simulink model "neupravljani_nelinearni_i_linearni_model"  (R2015a)
settings: Solver=ode4  StartTime=0.0  StopTime=700  FixedStep=0.01  RelTol=1e-3
values from neighbouring files (symbols this model uses):
  Ar1 = 0.04    [skript_drugi_deo.m]
  Ar2 = 0.04    [skript_drugi_deo.m]
  Cd1 = 0.65    [skript_drugi_deo.m]
  Cd2 = 0.65    [skript_drugi_deo.m]
  Cdh = 0.65    [skript_drugi_deo.m]
  df1_H1 = double(subs(df1_H1, [Uvh Uv2 H1 H2], [Uvh_N Uv2_N H1_N H2_N]))    [skript_drugi_deo.m]
  df1_Uvh = double(subs(df1_Uvh, [Uvh Uv2 H1 H2], [Uvh_N Uv2_N H1_N H2_N]))    [skript_drugi_deo.m]
  df2_H1 = double(subs(df2_H1, [Uvh Uv2 H1 H2], [Uvh_N Uv2_N H1_N H2_N]))    [skript_drugi_deo.m]
  df2_H2 = double(subs(df2_H2, [Uvh Uv2 H1 H2], [Uvh_N Uv2_N H1_N H2_N]))    [skript_drugi_deo.m]
  df2_Uv2 = double(subs(df2_Uv2, [Uvh Uv2 H1 H2], [Uvh_N Uv2_N H1_N H2_N]))    [skript_drugi_deo.m]
  g = 9.81    [skript_drugi_deo.m]
  H1_max = 1.5    [skript_drugi_deo.m]
  H1_min = 0    [skript_drugi_deo.m]
  H1_N = 0.7    [skript_drugi_deo.m]
  H2_max = 1.5    [skript_drugi_deo.m]
  H2_min = 0    [skript_drugi_deo.m]
  H2_N = 0.8    [skript_drugi_deo.m]
  Kv1 = 1.5/1000    (= 0.0015)    [skript_drugi_deo.m]
  Kv2 = 1.5/1000    (= 0.0015)    [skript_drugi_deo.m]
  Kvh = 1/1000    (= 0.001)    [skript_drugi_deo.m]
  Ph = 3.25*10^5    (= 325000)    [skript_drugi_deo.m]
  ro = 1000    [skript_drugi_deo.m]
  Uv1 = 3    [skript_drugi_deo.m]
  Uv2_max = 10    [skript_drugi_deo.m]
  Uv2_min = 0    [skript_drugi_deo.m]
  Uv2_N = double(solve(e2 == 0, U2_N))    [skript_drugi_deo.m]
  Uvh_max = 10    [skript_drugi_deo.m]
  Uvh_min = 0    [skript_drugi_deo.m]
  Uvh_N = double(solve(e1 == 0, Uh_N))    [skript_drugi_deo.m]
  w1 = 0.1    [skript_drugi_deo.m]
  w2 = 0.1    [skript_drugi_deo.m]
  wh = 0.03    [skript_drugi_deo.m]
settings Model: Creator=Nikola  LastModifiedBy=Nikola

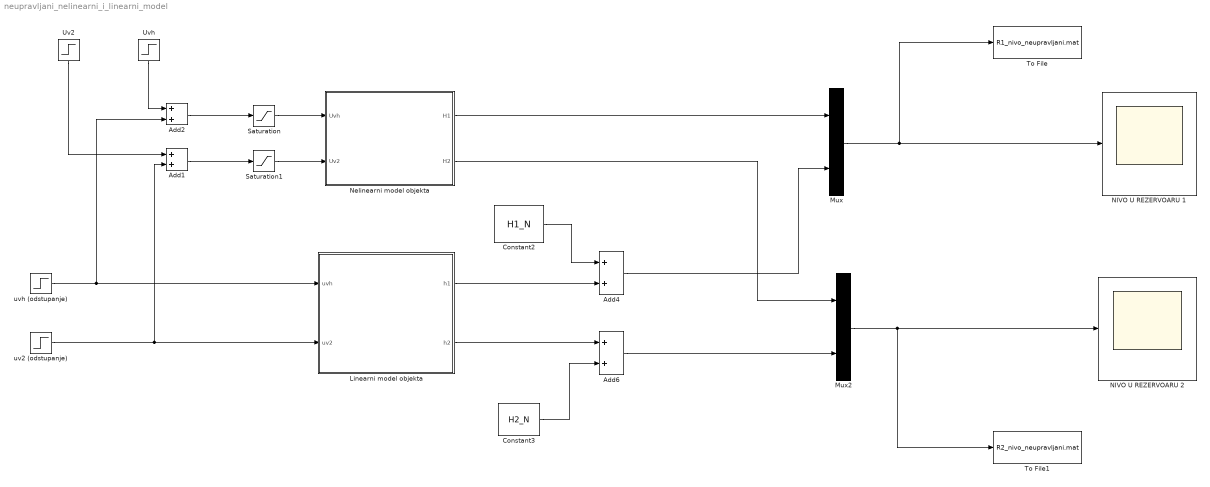
== system neupravljani_nelinearni_i_linearni_model ==
  Add{1..2,4,6} (4 alike) : Sum
  Constant2 : Constant  Value=H1_N
  Constant3 : Constant  Value=H2_N
  Linearni model objekta : Subsystem
  Mux : Mux  Inputs=2
  Mux2 : Mux  Inputs=2
  NIVO U REZERVOARU 1 : Scope
      settings: SaveName=ScopeData3
  NIVO U REZERVOARU 2 : Scope
      settings: SaveName=ScopeData4
  Nelinearni model objekta : Subsystem
  Saturation : Saturate  UpperLimit=Uvh_max  LowerLimit=Uvh_min
  Saturation1 : Saturate  UpperLimit=Uv2_max  LowerLimit=Uv2_min
  To File : ToFile  Filename=R1_nivo_neupravljani.mat  MatrixName=H1_neupravljani
  To File1 : ToFile  Filename=R2_nivo_neupravljani.mat  MatrixName=H2_neupravljani
  Uv2 : Step  Time=0  After=Uv2_N  SampleTime=0
  Uvh : Step  Time=0  After=Uvh_N  SampleTime=0
  uv2 (odstupanje) : Step  Time=0  After=0  SampleTime=0
  uvh (odstupanje) : Step  Time=150  After=0.1  SampleTime=0
  wires:
  Uvh/1 -> Add2/1
  Uv2/1 -> Add1/1
  Nelinearni model objekta/1(H1) -> Mux/1
  Mux/1 -> To File/1, NIVO U REZERVOARU 1/1
  Nelinearni model objekta/2(H2) -> Mux2/1
  Mux2/1 -> NIVO U REZERVOARU 2/1, To File1/1
  Add2/1 -> Saturation/1
  Add1/1 -> Saturation1/1
  uvh (odstupanje)/1 -> Linearni model objekta/1(uvh), Add2/2
  uv2 (odstupanje)/1 -> Linearni model objekta/2(uv2), Add1/2
  Linearni model objekta/1(h1) -> Add4/2
  Constant2/1 -> Add4/1
  Add4/1 -> Mux/2
  Add6/1 -> Mux2/2
  Linearni model objekta/2(h2) -> Add6/1
  Constant3/1 -> Add6/2
  Saturation/1 -> Nelinearni model objekta/1(Uvh)
  Saturation1/1 -> Nelinearni model objekta/2(Uv2)

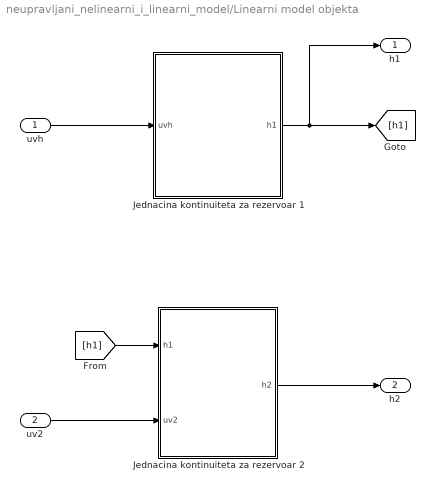
== system neupravljani_nelinearni_i_linearni_model/Linearni model objekta ==
  uvh : Inport
  uv2 : Inport  Port=2
  Jednacina kontinuiteta za rezervoar 1 : Subsystem
  Jednacina kontinuiteta za rezervoar 2 : Subsystem
  h1 : Outport
  h2 : Outport  Port=2
  wires:
  Jednacina kontinuiteta za rezervoar 1/1(h1) -> [h1], h1/1
  [h1] -> Jednacina kontinuiteta za rezervoar 2/1(h1)
  Jednacina kontinuiteta za rezervoar 2/1(h2) -> h2/1
  uvh/1 -> Jednacina kontinuiteta za rezervoar 1/1(uvh)
  uv2/1 -> Jednacina kontinuiteta za rezervoar 2/2(uv2)

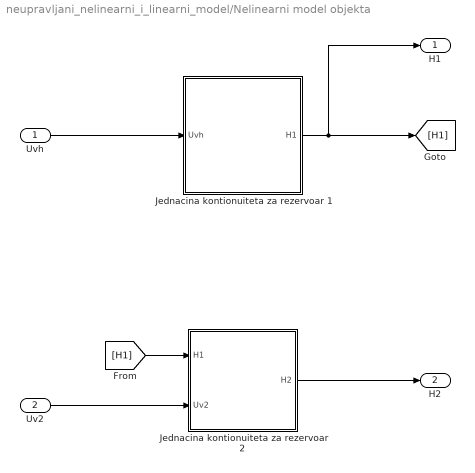
== system neupravljani_nelinearni_i_linearni_model/Nelinearni model objekta ==
  Uvh : Inport
  Uv2 : Inport  Port=2
  Jednacina kontionuiteta za rezervoar 1 : Subsystem
  Jednacina kontionuiteta za rezervoar 2 : Subsystem
  H1 : Outport
  H2 : Outport  Port=2
  wires:
  Jednacina kontionuiteta za rezervoar 1/1(H1) -> [H1], H1/1
  Uvh/1 -> Jednacina kontionuiteta za rezervoar 1/1(Uvh)
  Uv2/1 -> Jednacina kontionuiteta za rezervoar 2/2(Uv2)
  Jednacina kontionuiteta za rezervoar 2/1(H2) -> H2/1
  [H1] -> Jednacina kontionuiteta za rezervoar 2/1(H1)

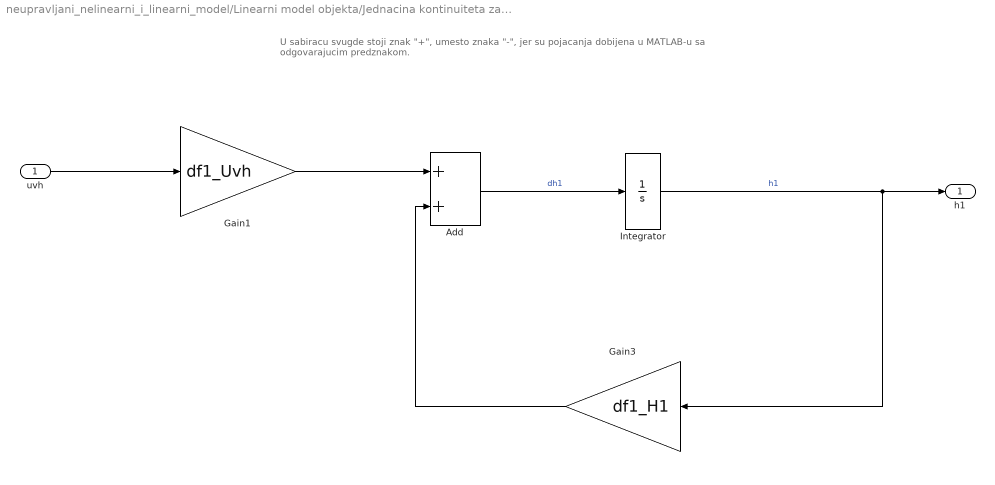
== system neupravljani_nelinearni_i_linearni_model/Linearni model objekta/Jednacina kontinuiteta za rezervoar 1 ==
  note: U sabiracu svugde stoji znak "+", umesto znaka "-", jer
      | su pojacanja dobijena u MATLAB-u sa
      | odgovarajucim predznakom.
  uvh : Inport
  Add : Sum
  Gain1 : Gain  Gain=df1_Uvh
  Gain3 : Gain  Gain=df1_H1
  Integrator : Integrator
  h1 : Outport
  wires:
  uvh/1 -> Gain1/1
  Add/1 -> Integrator/1  "dh1"
  Integrator/1 -> Gain3/1, h1/1  "h1"
  Gain3/1 -> Add/2
  Gain1/1 -> Add/1

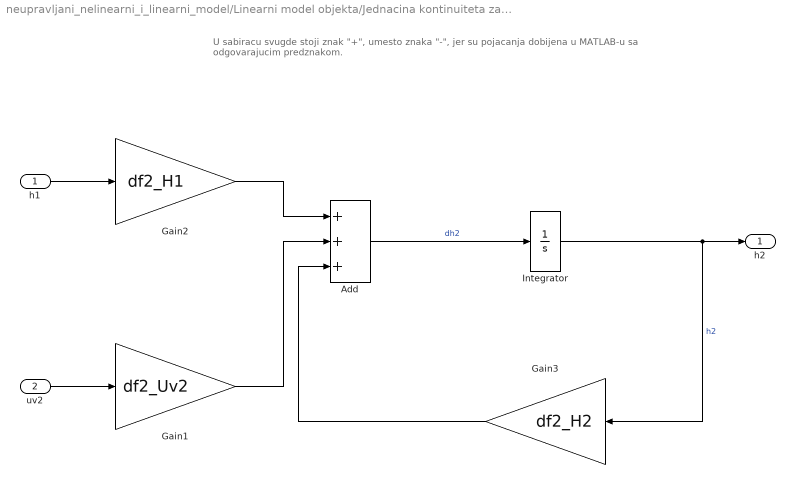
== system neupravljani_nelinearni_i_linearni_model/Linearni model objekta/Jednacina kontinuiteta za rezervoar 2 ==
  note: U sabiracu svugde stoji znak "+", umesto znaka "-", jer
      | su pojacanja dobijena u MATLAB-u sa
      | odgovarajucim predznakom.
  h1 : Inport
  uv2 : Inport  Port=2
  Add : Sum  Inputs=+++
  Gain1 : Gain  Gain=df2_Uv2
  Gain2 : Gain  Gain=df2_H1
  Gain3 : Gain  Gain=df2_H2
  Integrator : Integrator
  h2 : Outport
  wires:
  Add/1 -> Integrator/1  "dh2"
  h1/1 -> Gain2/1
  Gain2/1 -> Add/1
  uv2/1 -> Gain1/1
  Gain1/1 -> Add/2
  Integrator/1 -> Gain3/1, h2/1  "h2"
  Gain3/1 -> Add/3

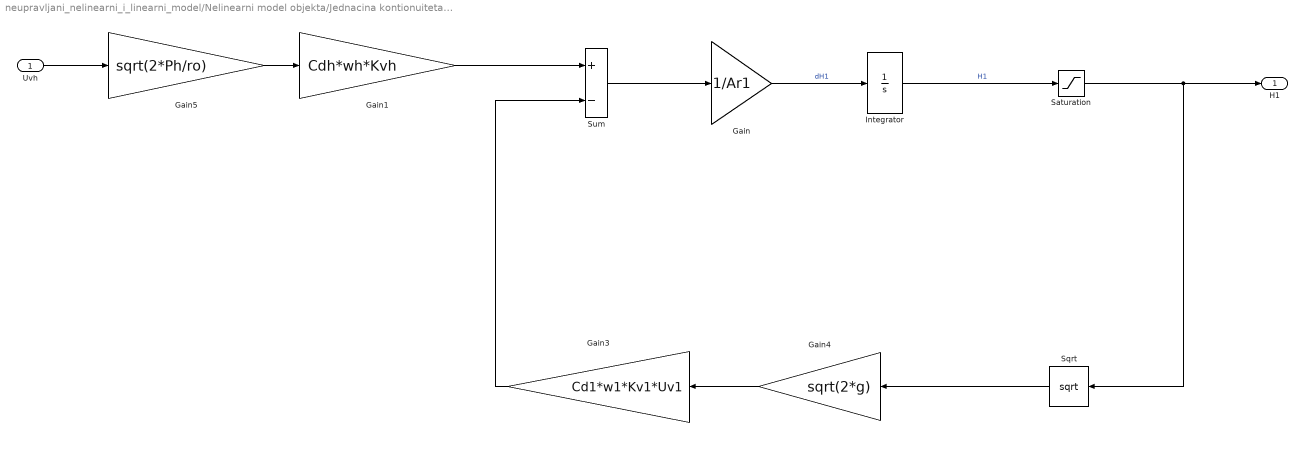
== system neupravljani_nelinearni_i_linearni_model/Nelinearni model objekta/Jednacina kontionuiteta za rezervoar 1 ==
  Uvh : Inport
  Gain : Gain  Gain=1/Ar1
  Gain1 : Gain  Gain=Cdh*wh*Kvh
  Gain3 : Gain  Gain=Cd1*w1*Kv1*Uv1
  Gain4 : Gain  Gain=sqrt(2*g)
  Gain5 : Gain  Gain=sqrt(2*Ph/ro)
  Integrator : Integrator  InitialCondition=H1_N
  Saturation : Saturate  UpperLimit=H1_max  LowerLimit=H1_min
  Sqrt : Sqrt  SaturateOnIntegerOverflow=on
  Sum : Sum  Inputs=+-
  H1 : Outport
  wires:
  Gain/1 -> Integrator/1  "dH1"
  Sum/1 -> Gain/1
  Integrator/1 -> Saturation/1  "H1"
  Sqrt/1 -> Gain4/1
  Gain4/1 -> Gain3/1
  Gain5/1 -> Gain1/1
  Uvh/1 -> Gain5/1
  Saturation/1 -> Sqrt/1, H1/1
  Gain3/1 -> Sum/2
  Gain1/1 -> Sum/1

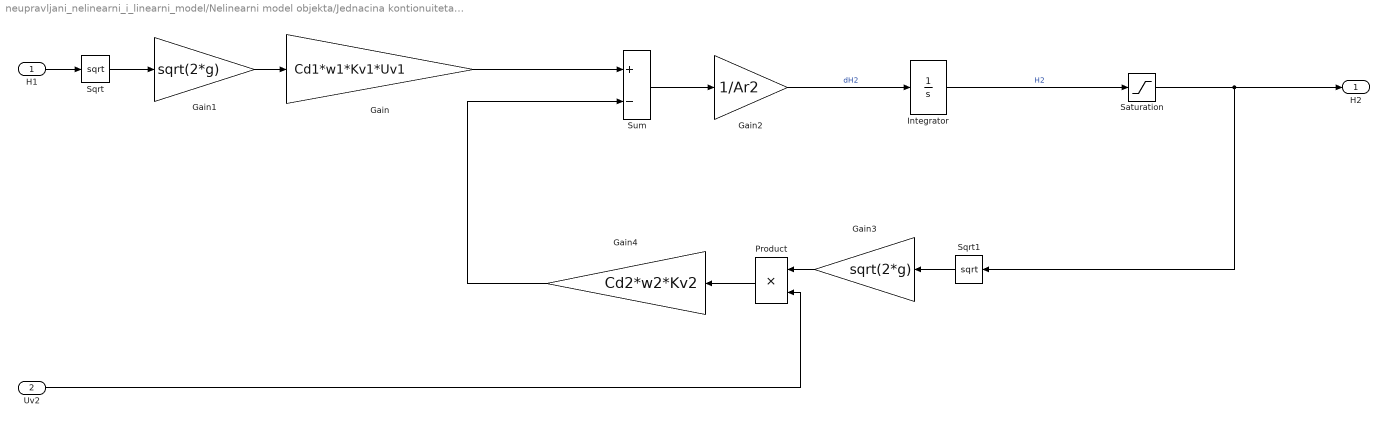
== system neupravljani_nelinearni_i_linearni_model/Nelinearni model objekta/Jednacina kontionuiteta za rezervoar 2 ==
  H1 : Inport
  Uv2 : Inport  Port=2
  Gain : Gain  Gain=Cd1*w1*Kv1*Uv1
  Gain1 : Gain  Gain=sqrt(2*g)
  Gain2 : Gain  Gain=1/Ar2
  Gain3 : Gain  Gain=sqrt(2*g)
  Gain4 : Gain  Gain=Cd2*w2*Kv2
  Integrator : Integrator  InitialCondition=H2_N
  Product : Product
  Saturation : Saturate  UpperLimit=H2_max  LowerLimit=H2_min
  Sqrt : Sqrt  SaturateOnIntegerOverflow=on
  Sqrt1 : Sqrt  SaturateOnIntegerOverflow=on
  Sum : Sum  Inputs=+-
  H2 : Outport
  wires:
  H1/1 -> Sqrt/1
  Sqrt/1 -> Gain1/1
  Gain1/1 -> Gain/1
  Gain/1 -> Sum/1
  Sum/1 -> Gain2/1
  Gain2/1 -> Integrator/1  "dH2"
  Integrator/1 -> Saturation/1  "H2"
  Sqrt1/1 -> Gain3/1
  Gain3/1 -> Product/1
  Uv2/1 -> Product/2
  Product/1 -> Gain4/1
  Gain4/1 -> Sum/2
  Saturation/1 -> Sqrt1/1, H2/1
